simulink model "benchmark_model_2"  (R2021a)
settings: Solver=ode1  StartTime=0.0  StopTime=Tend  FixedStep=0.0001  MaxStep=0.1  MinStep=0.0001  AbsTol=0.01  EnableMultiTasking=on
values from neighbouring files (symbols this model uses):
  A1 = 0.00017774967488    [engine_data.mat]
  A2 = 740220.330082    [engine_data.mat]
  AL = [6 6.5 7 7.5 8 8.5 9 9.5 10 10.5 11 11.5 ... (33 elements, 33x1)]    [engine_data.mat]
  AM0 = 0.02884    [engine_data.mat]
  AREA = 0.00580880481649    [engine_data.mat]
  BORE = 0.086    [engine_data.mat]
  C_EGR = 1.5    [engine_data.mat]
  c_f = 800000    [engine_data.mat]
  c_T = 1    [engine_data.mat]
  CAIR = [0 0 0 0.21 0 0 0.79]    [engine_data.mat]
  cCO = 0    [engine_data.mat]
  cCO2 = 0    [engine_data.mat]
  cH2 = 0    [engine_data.mat]
  cH2O = 0    [engine_data.mat]
  cHC = 0    [engine_data.mat]
  cN2 = 0.79    [engine_data.mat]
  CO = [22.3416398376 20.8398063107 19.3759939408 17.9445472871 16.538827802 15.1528221174 13.7819470707 12.4234138404 11.076283262 9.74128071245 8.42044156849 7.11667724438 ... (33 elements, 33x1)]    [engine_data.mat]
  CO2 = [1.08016197936 1.63070203699 2.20578946805 2.80905596198 3.44329822989 4.11013545224 4.80975559522 5.54078746844 6.30033629562 7.08419123341 7.88717005398 8.70352822078 ... (33 elements, 33x1)]    [engine_data.mat]
  cO2 = 0.21    [engine_data.mat]
  DEN0 = 1.17881164668    [engine_data.mat]
  EGR_dia = 0.02    [engine_data.mat]
  EGR_sk = 0.125663706144    [engine_data.mat]
  EX_AREA = 0.00137444678595    [engine_data.mat]
  EX_M_AR = 0.0258532162804    [engine_data.mat]
  EXO = 40    [engine_data.mat]
  FD0 = 5    [engine_data.mat]
  FOM = [12 11.348 6.233 5 5.449 8.523 5]    [engine_data.mat]
  FR0 = 0    [engine_data.mat]
  FR_C1 = 305.731    [engine_data.mat]
  FR_C2 = 1.70183    [engine_data.mat]
  FR_C3 = 3188.7424    [engine_data.mat]
  FR_C4 = 0.000296028194151    [engine_data.mat]
  FR_C5 = 1.03    [engine_data.mat]
  H2 = [17.3855302766 15.0102176452 12.8820660449 10.9850020715 9.30240027035 7.81790027685 6.51548255669 5.37933989743 4.39378660966 3.5433012035 2.8127075229 2.1874445405 ... (33 elements, 33x1)]    [engine_data.mat]
  H2O = [3.81120036781 5.32559240945 6.64944794012 7.79700886885 8.78142378855 9.61507632366 10.310008356 10.8782622871 11.3320540899 11.6837509075 11.9456809954 12.1298414055 ... (33 elements, 33x1)]    [engine_data.mat]
  HC = [5481.3024964 4476.06435729 3754.34247414 3215.30411383 2799.83726136 2471.30975971 2205.97110777 1987.83348465 1805.78690133 1651.89669698 1520.35918152 1406.8402103 ... (33 elements, 33x1)]    [engine_data.mat]
  INC = 0    [engine_data.mat]
  INO = -40    [engine_data.mat]
  KET = 0.001    [engine_data.mat]
  Kex = 1.28224854645    [engine_data.mat]
  Kh = 0.00462    [engine_data.mat]
  MAS0 = 0.00471524658673    [engine_data.mat]
  MCh = 0.000588883862304    [engine_data.mat]
  MHC = 0.01383448    [engine_data.mat]
  MN2 = 0.028    [engine_data.mat]
  MO2 = 0.032    [engine_data.mat]
  MOLcylT = 0.00157069204711    [engine_data.mat]
  N2 = [54.5020363032 56.4529864816 58.2465252261 59.8999246568 61.4284172656 62.8453054261 64.1621746691 65.3891205654 66.5349581592 67.6074047194 68.6132342687 69.5584035698 ... (33 elements, 33x1)]    [engine_data.mat]
  O2 = [0.331300985803 0.293088680307 0.264743132617 0.242930742419 0.225648917415 0.211629427842 0.200034641439 0.190292592782 0.182002893523 0.174881554044 0.168729672297 0.163420998081 ... (33 elements, 33x1)]    [engine_data.mat]
  PR0 = 101324.72    [engine_data.mat]
  R150 = 157.079632679    [engine_data.mat]
  Rabs = 8.31441    [engine_data.mat]
  SPEC = [4 0.086 0.086 0.043 0.14665 14 1 0.1 0 0.5 0.005 0 ... (19 elements, 19x1)]    [engine_data.mat]
  TBORE = 0.055    [engine_data.mat]
  Tend = 120    [engine_data.mat]
  Th_HC = 0.1    [engine_data.mat]
  Th_knock = 0.401961937891    [engine_data.mat]
  THEX = [0 1 2 3 4 5 6 7 8 9 10 11 ... (721 elements, 1x721)]    [engine_data.mat]
  THIN = [0 1 2 3 4 5 6 7 8 9 10 11 ... (721 elements, 1x721)]    [engine_data.mat]
  TM0 = 298.15    [engine_data.mat]
  Tstart = 5    [engine_data.mat]
  TW0 = 353.15    [engine_data.mat]
  V_EX = 0.0001    [engine_data.mat]
  VAREX = [0 0 0 0 0 0 0 0 0 0 0 0 ... (721 elements, 1x721)]    [engine_data.mat]
  VARIN = [0 0 0 0 0 0 0 0 0 0 0 0 ... (721 elements, 1x721)]    [engine_data.mat]
  VH = 0.000499557214218    [engine_data.mat]
  VT = 3.84274780168e-05    [engine_data.mat]
  WOM = [0.01383448 0.04401 0.02801 0.032 0.002016 0.018016 0.028]    [engine_data.mat]
  y = 1.81    [engine_data.mat]
undefined symbols (not defined in the file or in its folder): DiscIntNeverNeededParam
libraries: pid_lib x3
(part 1 of 7)
settings Model: SimulationMode=accelerator  ExtModeTrigMode=oneshot  ExtModeArmWhenConnect=off  Creator=mobile  LastModifiedBy=Seb
settings SolverCC: AutoScaleAbsTol=off  ZeroCrossControl=DisableAll  AlgebraicLoopSolver=TrustRegion
settings DataIOCC: SaveFormat=Array  SignalLoggingSaveFormat=ModelDataLogs  ReturnWorkspaceOutputs=off
settings OptimizationCC: BlockReduction=off  BooleanDataType=off  ExpressionDepthLimit=2147483647  InitFltsAndDblsToZero=on  LifeSpan=inf
settings DebuggingCC: SaveWithParameterizedLinksMsg=none  UnderspecifiedInitializationDetection=Classic  MergeDetectMultiDrivingBlocksExec=none  SignalResolutionControl=TryResolveAllWithWarning  MultiTaskDSMMsg=warning  MultiTaskCondExecSysMsg=none  IntegerOverflowMsg=none  FcnCallInpInsideContextMsg=warning  StateNameClashWarn=warning  SFUnexpectedBacktrackingDiag=warning  SFNoUnconditionalDefaultTransitionDiag=warning  SFExecutionAtInitializationDiag=none  SFMachineParentedDataDiag=warning  IntegerSaturationMsg=none  ArithmeticOperatorsInVariantConditions=warning
settings HardwareCC: ProdBitPerPointer=32  ProdBitPerSizeT=32  ProdBitPerPtrDiffT=32  ProdLargestAtomicFloat=None  ProdIntDivRoundTo=Undefined  ProdEndianess=Unspecified  ProdWordSize=32  ProdHWDeviceType=32-bit Generic  TargetBitPerPointer=64  TargetBitPerSizeT=64  TargetBitPerPtrDiffT=64  TargetLongLongMode=on  TargetIntDivRoundTo=Zero  TargetEndianess=LittleEndian  TargetWordSize=64  TargetHWDeviceType=MATLAB Host  ProdEqTarget=off
settings ModelReferenceCC: PropagateSignalLabelsOutOfModel=off
settings SFSimCC: SimUseLocalCustomCode=off  CustomCodeUndefinedFunction=UseInterfaceOnly
settings RTWCC: RTWUseLocalCustomCode=off
settings CodeAppCC: StateflowObjectComments=on
settings GRTTargetCC: TargetFcnLib=ansi_tfl_tmw.mat  TargetLangStandard=C89/C90 (ANSI)  CombineOutputUpdateFcns=off  GRTInterface=on
settings ConfigComp: CovMetricSettings=dw  CovSaveCumulativeToWorkspaceVar=on  CovSaveSingleToWorkspaceVar=on  CovExternalEMLEnable=off

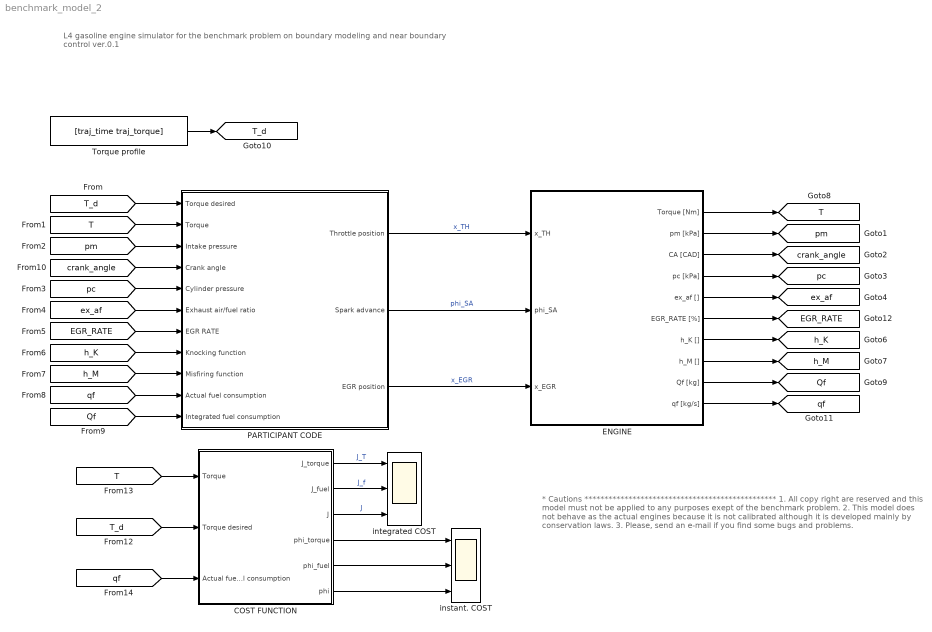
== system benchmark_model_2 ==
  note: * Cautions ************************************************
      | 1. All copy right are reserved and this model must not be applied to
      |     any purposes exept of the benchmark problem.
      | 2. This model does not behave as the actual engines because it is not
      |     calibrated although it is developed mainly by conservation laws.
      | 3. Please, send an e-mail if you find some bugs and problems.
  note: L4 gasoline engine simulator for the benchmark problem
      | on boundary modeling and near boundary control ver.0.1
  COST FUNCTION : Subsystem
  ENGINE : Subsystem
  PARTICIPANT CODE : Subsystem
  Torque profile : FromWorkspace  VariableName=[traj_time traj_torque]  SampleTime=-1  OutputAfterFinalValue=Holding final value
  instant. COST : Scope  NumInputPorts=3
  integrated COST : Scope  NumInputPorts=3
  tag scope: EGR_RATE=global, Qf=global, T=global, T_d=global, crank_angle=global, ex_af=global, h_K=global, h_M=global, pc=global, pm=global, qf=global
  wires:
  [EGR_RATE] -> PARTICIPANT CODE/7(EGR RATE)
  [h_M] -> PARTICIPANT CODE/9(Misfiring function)
  [pc] -> PARTICIPANT CODE/5(Cylinder pressure)
  [h_K] -> PARTICIPANT CODE/8(Knocking function)
  [T] -> PARTICIPANT CODE/2(Torque)
  [pm] -> PARTICIPANT CODE/3(Intake pressure)
  [qf] -> PARTICIPANT CODE/10(Actual fuel consumption)
  [ex_af] -> PARTICIPANT CODE/6(Exhaust air/fuel ratio)
  [Qf] -> PARTICIPANT CODE/11(Integrated fuel consumption)
  [T_d] -> PARTICIPANT CODE/1(Torque desired)
  Torque profile/1 -> [T_d]
  COST FUNCTION/1(J_torque) -> integrated COST/1  "J_T"
  COST FUNCTION/2(J_fuel) -> integrated COST/2  "J_f"
  COST FUNCTION/3(J) -> integrated COST/3  "J"
  [T] -> COST FUNCTION/1(Torque)
  [T_d] -> COST FUNCTION/2(Torque desired)
  [qf] -> COST FUNCTION/3(Actual fuel consumption)
  [crank_angle] -> PARTICIPANT CODE/4(Crank angle)
  PARTICIPANT CODE/1(Throttle position) -> ENGINE/1(x_TH)  "x_TH"
  PARTICIPANT CODE/2(Spark advance) -> ENGINE/2(phi_SA)  "phi_SA"
  PARTICIPANT CODE/3(EGR position) -> ENGINE/3(x_EGR)  "x_EGR"
  ENGINE/2(pm [kPa]) -> [pm]
  ENGINE/3(CA [CAD]) -> [crank_angle]
  ENGINE/4(pc [kPa]) -> [pc]
  ENGINE/5(ex_af []) -> [ex_af]
  ENGINE/7(h_K []) -> [h_K]
  ENGINE/8(h_M []) -> [h_M]
  ENGINE/1(Torque [Nm]) -> [T]
  ENGINE/9(Qf [kg]) -> [Qf]
  ENGINE/10(qf [kg/s]) -> [qf]
  ENGINE/6(EGR_RATE [%]) -> [EGR_RATE]
  COST FUNCTION/4(phi_torque) -> instant. COST/1
  COST FUNCTION/5(phi_fuel) -> instant. COST/2
  COST FUNCTION/6(phi) -> instant. COST/3

== system benchmark_model_2/COST FUNCTION ==
  Torque : Inport
  Torque desired : Inport  Port=2
  Actual fuel consumption : Inport  Port=3
  Add : Sum  Inputs=+-
  Add1 : Sum
  Add2 : Sum
  Gain : Gain  Gain=c_f
  Gain1 : Gain  Gain=c_T
  Gain2 : Gain  Gain=c_f
  Gain3 : Gain  Gain=c_T
  Integrator : Integrator
  Integrator1 : Integrator
  Math Function : Math  Operator=square  SignedPower=on  SaturateOnIntegerOverflow=on
  Product : Product
  Product1 : Product
  Step : Step  Time=Tstart  SampleTime=0
  J_torque : Outport
  J_fuel : Outport  Port=2
  J : Outport  Port=3
  phi_torque : Outport  Port=4
  phi_fuel : Outport  Port=5
  phi : Outport  Port=6
  wires:
  Torque/1 -> Add/1
  Torque desired/1 -> Add/2
  Gain/1 -> Add1/2, J_fuel/1
  Gain1/1 -> Add1/1, J_torque/1
  Math Function/1 -> Gain3/1, Integrator/1
  Integrator/1 -> Gain1/1
  Actual fuel consumption/1 -> Product/1
  Product/1 -> Gain2/1, Integrator1/1
  Step/1 -> Product1/2, Product/2
  Add/1 -> Product1/1
  Product1/1 -> Math Function/1
  Add1/1 -> J/1
  Integrator1/1 -> Gain/1
  Gain3/1 -> phi_torque/1, Add2/1
  Add2/1 -> phi/1
  Gain2/1 -> Add2/2, phi_fuel/1

== system benchmark_model_2/ENGINE ==
  x_TH : Inport
  phi_SA : Inport  Port=2
  x_EGR : Inport  Port=3
  Changing units : Subsystem
  EGR%2Lift : Fcn  Expr=u(1)/100*0.125*EGR_dia
  Ground1 : Ground
  Product : Product  RndMeth=Zero
  Terminator{,1..3} (4 alike) : Terminator
  Torq2VVT : Lookup_n-D  NumberOfTableDimensions=1  BreakpointsForDimension1=[0,6,10,20,180]  Table=[10,5,0,0,0]  RndMeth=Simplest  InputSameDT=on
  V2Vec : Constant  Value=[1 1 1 1]
  engine_s : Subsystem
  rpm : Constant  Value=1500
  Torque [Nm] : Outport
  pm [kPa] : Outport  Port=2
  CA [CAD] : Outport  Port=3
  pc [kPa] : Outport  Port=4
  ex_af [] : Outport  Port=5
  EGR_RATE [%] : Outport  Port=6
  h_K [] : Outport  Port=7
  h_M [] : Outport  Port=8
  Qf [kg] : Outport  Port=9
  qf [kg/s] : Outport  Port=10
  wires:
  engine_s/7(EGR) -> Changing units/5(C_rate)
  engine_s/6(pm) -> Changing units/4(pm)
  engine_s/10(M_HC) -> Changing units/8(RH)
  engine_s/8(R_KC) -> Changing units/6(R_KC)
  engine_s/9(B_KC) -> Changing units/7(B_KC)
  engine_s/11(TR) -> Changing units/9(torque)
  engine_s/12(Qf) -> Changing units/10(Qf)
  Ground1/1 -> engine_s/4(ECU_fi)
  engine_s/1(rps) -> Terminator/1
  engine_s/2(mt) -> Terminator1/1
  Torq2VVT/1 -> engine_s/1(ECU_VVT)
  EGR%2Lift/1 -> engine_s/5(ECU_EGR)
  Product/1 -> engine_s/3(ECU_sa)
  V2Vec/1 -> Product/2
  phi_SA/1 -> Product/1
  x_EGR/1 -> EGR%2Lift/1
  x_TH/1 -> engine_s/2(ECU_dth)
  engine_s/13(qf) -> Changing units/11(qf)
  Changing units/2(pm [kPa]) -> pm [kPa]/1
  Changing units/3(crank_angle [deg]) -> CA [CAD]/1
  Changing units/4(pc [kpa]) -> pc [kPa]/1
  Changing units/5(ex_af) -> ex_af []/1
  Changing units/12(qf [kg/s]) -> qf [kg/s]/1
  Changing units/11(Qf [kg]) -> Qf [kg]/1
  Changing units/10(T [Nm]) -> Torque [Nm]/1
  Changing units/9(h_M) -> h_M []/1
  Changing units/8(h_K) -> h_K []/1
  Changing units/6(EGR [%]) -> EGR_RATE [%]/1
  [T_d] -> Torq2VVT/1
  rpm/1 -> Changing units/12(rpm), engine_s/6(rpm)
  engine_s/4(afm) -> Changing units/2(af)
  engine_s/5(pc) -> Changing units/3(pc)
  engine_s/3(st) -> Changing units/1(st)
  Changing units/1(RPM) -> Terminator3/1
  Changing units/7(I_K) -> Terminator2/1

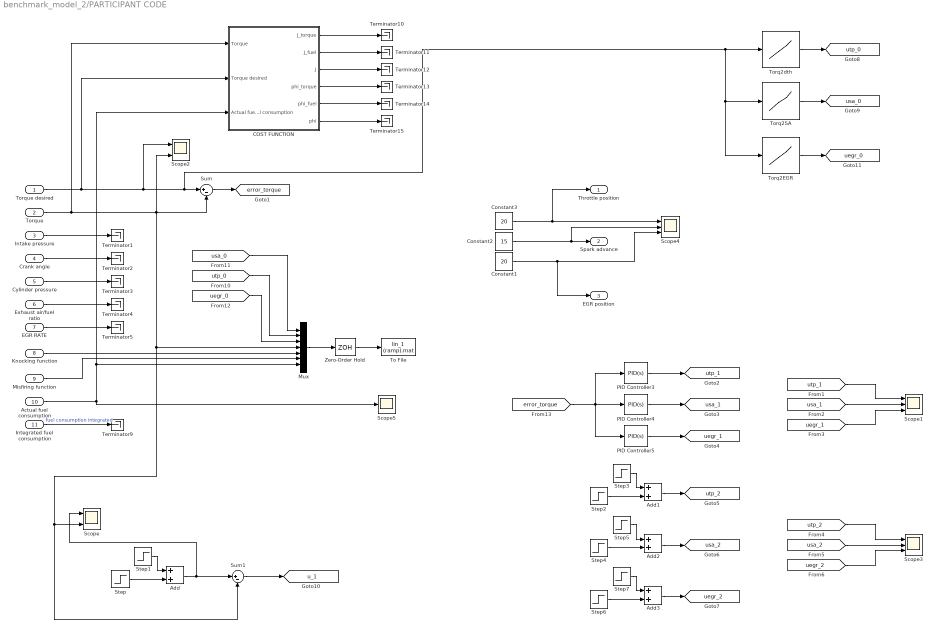
== system benchmark_model_2/PARTICIPANT CODE ==
  Torque desired : Inport
  Torque : Inport  Port=2
  Intake pressure : Inport  Port=3
  Crank angle : Inport  Port=4
  Cylinder pressure : Inport  Port=5
  Exhaust air/fuel ratio : Inport  Port=6
  EGR RATE : Inport  Port=7
  Knocking function : Inport  Port=8
  Misfiring function : Inport  Port=9
  Actual fuel consumption : Inport  Port=10
  Integrated fuel consumption : Inport  Port=11
  Add{,1..3} (4 alike) : Sum
  COST FUNCTION : Subsystem
  Constant1 : Constant  Value=20
  Constant2 : Constant  Value=15
  Constant3 : Constant  Value=20
  Mux : Mux  Inputs=7
  PID Controller3 : pid_lib/PID Controller  Controller=PID  Form=Parallel  TimeDomain=Continuous-time  UseExternalTs=off  SampleTime=-1  IntegratorMethod=Forward Euler  FilterMethod=Forward Euler  ControllerParametersSource=internal  P=0.15  I=0.75  D=0  UseFilter=on  N=100  TunerSelectOption=Transfer Function Based (PID Tuner App)  InitialConditionSource=internal  InitialConditionForIntegrator=0  InitialConditionForFilter=0  DifferentiatorICPrevScaledInput=0  ExternalReset=none  TrackingMode=off  Kt=1  LimitOutput=off  SatLimitsSource=internal  UpperSaturationLimit=inf  LowerSaturationLimit=-inf  LinearizeAsGain=on  AntiWindupMode=none  Kb=1  POutMin=[]  POutMax=[]  IOutMin=[]  IOutMax=[]  DOutMin=[]  DOutMax=[]  NOutMin=[]  NOutMax=[]  SumOutMin=[]  SumOutMax=[]  SaturationOutMin=[]  SaturationOutMax=[]  PParamMin=[]  PParamMax=[]  IParamMin=[]  IParamMax=[]  DParamMin=[]  DParamMax=[]  NParamMin=[]  NParamMax=[]  KbParamMin=[]  KbParamMax=[]  KtParamMin=[]  KtParamMax=[]  KbOutMin=[]  KbOutMax=[]  KtOutMin=[]  KtOutMax=[]  IntegratorOutMin=[]  IntegratorOutMax=[]  FilterOutMin=[]  FilterOutMax=[]  SumI1OutMin=[]  SumI1OutMax=[]  SumI2OutMin=[]  SumI2OutMax=[]  SumI3OutMin=[]  SumI3OutMax=[]  SumI4OutMin=[]  SumI4OutMax=[]  SumDOutMin=[]  SumDOutMax=[]  DifferentiatorOutMin=[]  DifferentiatorOutMax=[]  FilterDiffOutCoefMin=[]  FilterDiffOutCoefMax=[]  ReciprocalOutMin=[]  ReciprocalOutMax=[]  SumDenOutMin=[]  SumDenOutMax=[]  SumNumOutMin=[]  SumNumOutMax=[]  DivideOutMin=[]  DivideOutMax=[]  UdiffTsProdOutMin=[]  UdiffTsProdOutMax=[]  NTsProdOutMin=[]  NTsProdOutMax=[]  UintegralTsProdOutMin=[]  UintegralTsProdOutMax=[]  UngainTsProdOutMin=[]  UngainTsProdOutMax=[]  IntegratorContinuousStateAttributes=''  IntegratorStateMustResolveToSignalObject=off  IntegratorRTWStateStorageClass=Auto  FilterContinuousStateAttributes=''  FilterStateMustResolveToSignalObject=off  FilterRTWStateStorageClass=Auto  ParallelPVariant=InternalParameters  IdealPVariant=Disabled  IVariant=InternalParameters  DVariant=InternalParameters  IntegratorVariant=Continuous  SatVariant=Disabled  AWVariant=Passthrough  PCopyVariant=Disabled  TRVariant=Disabled  FdbkBlocksVariant=Forward  IdealPFdbkVariant=Disabled  SatFdbkVariant=Disabled  DerivativeFilterVariant=ContFilter  NVariant=InternalParameters  NCopyVariant=Disabled  FilterICVariant=InternalICsFilter  IntegratorICVariant=InternalICs  ExternalResetVariant=Disabled  TRSumVariant=Passthrough  SumFdbkVariant=Disabled  SumVariant=Sum_PID  TsampFilterVariant=InternalTs  TsampNgainVariant=Passthrough  TsampIntegralVariant=Passthrough  ExternalSaturationOutDataTypeStr=Inherit: Same as second input
  PID Controller4 : pid_lib/PID Controller  Controller=PID  Form=Parallel  TimeDomain=Continuous-time  UseExternalTs=off  SampleTime=-1  IntegratorMethod=Forward Euler  FilterMethod=Forward Euler  ControllerParametersSource=internal  P=0.3  I=0.1  D=0  UseFilter=on  N=100  TunerSelectOption=Transfer Function Based (PID Tuner App)  InitialConditionSource=internal  InitialConditionForIntegrator=0  InitialConditionForFilter=0  DifferentiatorICPrevScaledInput=0  ExternalReset=none  TrackingMode=off  Kt=1  LimitOutput=off  SatLimitsSource=internal  UpperSaturationLimit=inf  LowerSaturationLimit=-inf  LinearizeAsGain=on  AntiWindupMode=none  Kb=1  POutMin=[]  POutMax=[]  IOutMin=[]  IOutMax=[]  DOutMin=[]  DOutMax=[]  NOutMin=[]  NOutMax=[]  SumOutMin=[]  SumOutMax=[]  SaturationOutMin=[]  SaturationOutMax=[]  PParamMin=[]  PParamMax=[]  IParamMin=[]  IParamMax=[]  DParamMin=[]  DParamMax=[]  NParamMin=[]  NParamMax=[]  KbParamMin=[]  KbParamMax=[]  KtParamMin=[]  KtParamMax=[]  KbOutMin=[]  KbOutMax=[]  KtOutMin=[]  KtOutMax=[]  IntegratorOutMin=[]  IntegratorOutMax=[]  FilterOutMin=[]  FilterOutMax=[]  SumI1OutMin=[]  SumI1OutMax=[]  SumI2OutMin=[]  SumI2OutMax=[]  SumI3OutMin=[]  SumI3OutMax=[]  SumI4OutMin=[]  SumI4OutMax=[]  SumDOutMin=[]  SumDOutMax=[]  DifferentiatorOutMin=[]  DifferentiatorOutMax=[]  FilterDiffOutCoefMin=[]  FilterDiffOutCoefMax=[]  ReciprocalOutMin=[]  ReciprocalOutMax=[]  SumDenOutMin=[]  SumDenOutMax=[]  SumNumOutMin=[]  SumNumOutMax=[]  DivideOutMin=[]  DivideOutMax=[]  UdiffTsProdOutMin=[]  UdiffTsProdOutMax=[]  NTsProdOutMin=[]  NTsProdOutMax=[]  UintegralTsProdOutMin=[]  UintegralTsProdOutMax=[]  UngainTsProdOutMin=[]  UngainTsProdOutMax=[]  IntegratorContinuousStateAttributes=''  IntegratorStateMustResolveToSignalObject=off  IntegratorRTWStateStorageClass=Auto  FilterContinuousStateAttributes=''  FilterStateMustResolveToSignalObject=off  FilterRTWStateStorageClass=Auto  ParallelPVariant=InternalParameters  IdealPVariant=Disabled  IVariant=InternalParameters  DVariant=InternalParameters  IntegratorVariant=Continuous  SatVariant=Disabled  AWVariant=Passthrough  PCopyVariant=Disabled  TRVariant=Disabled  FdbkBlocksVariant=Forward  IdealPFdbkVariant=Disabled  SatFdbkVariant=Disabled  DerivativeFilterVariant=ContFilter  NVariant=InternalParameters  NCopyVariant=Disabled  FilterICVariant=InternalICsFilter  IntegratorICVariant=InternalICs  ExternalResetVariant=Disabled  TRSumVariant=Passthrough  SumFdbkVariant=Disabled  SumVariant=Sum_PID  TsampFilterVariant=InternalTs  TsampNgainVariant=Passthrough  TsampIntegralVariant=Passthrough  ExternalSaturationOutDataTypeStr=Inherit: Same as second input
  PID Controller5 : pid_lib/PID Controller  Controller=PID  Form=Parallel  TimeDomain=Continuous-time  UseExternalTs=off  SampleTime=-1  IntegratorMethod=Forward Euler  FilterMethod=Forward Euler  ControllerParametersSource=internal  P=0  I=0  D=0  UseFilter=on  N=100  TunerSelectOption=Transfer Function Based (PID Tuner App)  InitialConditionSource=internal  InitialConditionForIntegrator=0  InitialConditionForFilter=0  DifferentiatorICPrevScaledInput=0  ExternalReset=none  TrackingMode=off  Kt=1  LimitOutput=off  SatLimitsSource=internal  UpperSaturationLimit=inf  LowerSaturationLimit=-inf  LinearizeAsGain=on  AntiWindupMode=none  Kb=1  POutMin=[]  POutMax=[]  IOutMin=[]  IOutMax=[]  DOutMin=[]  DOutMax=[]  NOutMin=[]  NOutMax=[]  SumOutMin=[]  SumOutMax=[]  SaturationOutMin=[]  SaturationOutMax=[]  PParamMin=[]  PParamMax=[]  IParamMin=[]  IParamMax=[]  DParamMin=[]  DParamMax=[]  NParamMin=[]  NParamMax=[]  KbParamMin=[]  KbParamMax=[]  KtParamMin=[]  KtParamMax=[]  KbOutMin=[]  KbOutMax=[]  KtOutMin=[]  KtOutMax=[]  IntegratorOutMin=[]  IntegratorOutMax=[]  FilterOutMin=[]  FilterOutMax=[]  SumI1OutMin=[]  SumI1OutMax=[]  SumI2OutMin=[]  SumI2OutMax=[]  SumI3OutMin=[]  SumI3OutMax=[]  SumI4OutMin=[]  SumI4OutMax=[]  SumDOutMin=[]  SumDOutMax=[]  DifferentiatorOutMin=[]  DifferentiatorOutMax=[]  FilterDiffOutCoefMin=[]  FilterDiffOutCoefMax=[]  ReciprocalOutMin=[]  ReciprocalOutMax=[]  SumDenOutMin=[]  SumDenOutMax=[]  SumNumOutMin=[]  SumNumOutMax=[]  DivideOutMin=[]  DivideOutMax=[]  UdiffTsProdOutMin=[]  UdiffTsProdOutMax=[]  NTsProdOutMin=[]  NTsProdOutMax=[]  UintegralTsProdOutMin=[]  UintegralTsProdOutMax=[]  UngainTsProdOutMin=[]  UngainTsProdOutMax=[]  IntegratorContinuousStateAttributes=''  IntegratorStateMustResolveToSignalObject=off  IntegratorRTWStateStorageClass=Auto  FilterContinuousStateAttributes=''  FilterStateMustResolveToSignalObject=off  FilterRTWStateStorageClass=Auto  ParallelPVariant=InternalParameters  IdealPVariant=Disabled  IVariant=InternalParameters  DVariant=InternalParameters  IntegratorVariant=Continuous  SatVariant=Disabled  AWVariant=Passthrough  PCopyVariant=Disabled  TRVariant=Disabled  FdbkBlocksVariant=Forward  IdealPFdbkVariant=Disabled  SatFdbkVariant=Disabled  DerivativeFilterVariant=ContFilter  NVariant=InternalParameters  NCopyVariant=Disabled  FilterICVariant=InternalICsFilter  IntegratorICVariant=InternalICs  ExternalResetVariant=Disabled  TRSumVariant=Passthrough  SumFdbkVariant=Disabled  SumVariant=Sum_PID  TsampFilterVariant=InternalTs  TsampNgainVariant=Passthrough  TsampIntegralVariant=Passthrough  ExternalSaturationOutDataTypeStr=Inherit: Same as second input
  Scope : Scope  NumInputPorts=2
  Scope1 : Scope  NumInputPorts=3
  Scope2 : Scope  NumInputPorts=2
  Scope3 : Scope  NumInputPorts=3
  Scope4 : Scope  NumInputPorts=3
  Scope5 : Scope
  Step : Step  Time=0  After=50  SampleTime=0
  Step1 : Step  Time=15  After=30  SampleTime=0
  Step2 : Step  Time=Tend/3  Before=15  After=10  SampleTime=0
  Step3 : Step  Time=2*Tend/3  After=10  SampleTime=0
  Step4 : Step  Time=0  After=6  SampleTime=0
  Step5 : Step  Time=Tend/4  After=-4  SampleTime=0
  Step6 : Step  Time=0  After=0  SampleTime=0
  Step7 : Step  Time=3*Tend/4  After=5  SampleTime=0
  Sum : Sum  Inputs=|+-
  Sum1 : Sum  Inputs=|+-
  Terminator{1..5,9..15} (12 alike) : Terminator
  To File : ToFile  Filename=lin_1 (ramp).mat  MatrixName=u_y  SampleTime=0.1
  Torq2EGR : Lookup_n-D  NumberOfTableDimensions=1  BreakpointsForDimension1=[0,20,40,60,80,90,100,120,140,160,180,190]  Table=[0,0,2,5,10,18,25,20,14,9,5,2]  RndMeth=Simplest  InputSameDT=on
  Torq2SA : Lookup_n-D  NumberOfTableDimensions=1  BreakpointsForDimension1=[0,20,40,60,80,100,120,140,160,180]  Table=[20,25,25,25,18,14,14,14,14,14]  RndMeth=Simplest  InputSameDT=on
  Torq2dth : Lookup_n-D  NumberOfTableDimensions=1  BreakpointsForDimension1=[0,20,40,60,80,90,100,120,140,160,180,190]  Table=[7,9.2,10.8,12.6,15.4,18.2,23,25,27,29.5,35,36]  RndMeth=Simplest  InputSameDT=on
  Zero-Order Hold : ZeroOrderHold  SampleTime=0.1
  Throttle position : Outport
  Spark advance : Outport  Port=2
  EGR position : Outport  Port=3
  tag scope: error_torque=global, u_1=global, uegr_0=global, uegr_1=global, uegr_2=global, usa_0=global, usa_1=global, usa_2=global, utp_0=global, utp_1=global, utp_2=global
  wires:
  Torque desired/1 -> Scope2/1, Torq2EGR/1, Torq2SA/1, Torq2dth/1, Sum/1, COST FUNCTION/2(Torque desired)
  Integrated fuel consumption/1 -> Terminator9/1  "fuel consumption integrated"
  Torque/1 -> Sum/2, Scope/2, Sum1/2, Mux/4, Scope2/2, COST FUNCTION/1(Torque)
  Intake pressure/1 -> Terminator1/1
  Crank angle/1 -> Terminator2/1
  Cylinder pressure/1 -> Terminator3/1
  Exhaust air/fuel ratio/1 -> Terminator4/1
  EGR RATE/1 -> Terminator5/1
  Knocking function/1 -> Mux/5
  Misfiring function/1 -> Mux/6
  Actual fuel consumption/1 -> Scope5/1, COST FUNCTION/3(Actual fuel consumption), Mux/7
  COST FUNCTION/1(J_torque) -> Terminator10/1
  COST FUNCTION/2(J_fuel) -> Terminator11/1
  COST FUNCTION/3(J) -> Terminator12/1
  COST FUNCTION/4(phi_torque) -> Terminator13/1
  COST FUNCTION/5(phi_fuel) -> Terminator14/1
  COST FUNCTION/6(phi) -> Terminator15/1
  Step1/1 -> Add/1
  Step/1 -> Add/2
  Add/1 -> Scope/1, Sum1/1
  Sum1/1 -> [u_1]
  Sum/1 -> [error_torque]
  [error_torque] -> PID Controller4/1, PID Controller5/1, PID Controller3/1
  PID Controller3/1 -> [utp_1]
  PID Controller4/1 -> [usa_1]
  PID Controller5/1 -> [uegr_1]
  [uegr_1] -> Scope1/3
  [usa_1] -> Scope1/2
  [utp_1] -> Scope1/1
  Step2/1 -> Add1/2
  Step3/1 -> Add1/1
  Step5/1 -> Add2/1
  Step4/1 -> Add2/2
  Step6/1 -> Add3/2
  Add1/1 -> [utp_2]
  Add2/1 -> [usa_2]
  Add3/1 -> [uegr_2]
  Step7/1 -> Add3/1
  [utp_2] -> Scope3/1
  [usa_2] -> Scope3/2
  [uegr_2] -> Scope3/3
  Mux/1 -> Zero-Order Hold/1
  [uegr_0] -> Mux/3
  [utp_0] -> Mux/2
  [usa_0] -> Mux/1
  Torq2dth/1 -> [utp_0]
  Torq2SA/1 -> [usa_0]
  Torq2EGR/1 -> [uegr_0]
  Zero-Order Hold/1 -> To File/1
  Constant3/1 -> Throttle position/1, Scope4/1
  Constant2/1 -> Scope4/2, Spark advance/1
  Constant1/1 -> EGR position/1, Scope4/3

== system benchmark_model_2/ENGINE/Changing units ==
  st : Inport
  af : Inport  Port=2
  pc : Inport  Port=3
  pm : Inport  Port=4
  C_rate : Inport  Port=5
  R_KC : Inport  Port=6
  B_KC : Inport  Port=7
  RH : Inport  Port=8
  torque : Inport  Port=9
  Qf : Inport  Port=10
  qf : Inport  Port=11
  rpm : Inport  Port=12
  Gain : Gain  Gain=1/1000  SaturateOnIntegerOverflow=on  OutDataTypeStr=Inherit: Same as input  ParamDataTypeStr=Inherit: Same as input
  Gain2 : Gain  Gain=1.0e-3  SaturateOnIntegerOverflow=on  OutDataTypeStr=Inherit: Same as input  ParamDataTypeStr=Inherit: Same as input
  Gain3 : Gain  Gain=100  SaturateOnIntegerOverflow=on  OutDataTypeStr=Inherit: Same as input  ParamDataTypeStr=Inherit: Same as input
  select : Subsystem
  RPM : Outport
  pm [kPa] : Outport  Port=2
  crank_angle [deg] : Outport  Port=3
  pc [kpa] : Outport  Port=4
  ex_af : Outport  Port=5
  EGR [%] : Outport  Port=6
  I_K : Outport  Port=7
  h_K : Outport  Port=8
  h_M : Outport  Port=9
  T [Nm] : Outport  Port=10
  Qf [kg] : Outport  Port=11
  qf [kg/s] : Outport  Port=12
  wires:
  pm/1 -> Gain/1
  Gain/1 -> pm [kPa]/1
  pc/1 -> Gain2/1
  Gain2/1 -> pc [kpa]/1
  st/1 -> select/1(st)
  select/1(crank) -> crank_angle [deg]/1
  af/1 -> ex_af/1
  C_rate/1 -> Gain3/1
  Gain3/1 -> EGR [%]/1
  RH/1 -> h_M/1
  B_KC/1 -> h_K/1
  R_KC/1 -> I_K/1
  rpm/1 -> RPM/1
  torque/1 -> T [Nm]/1
  Qf/1 -> Qf [kg]/1
  qf/1 -> qf [kg/s]/1

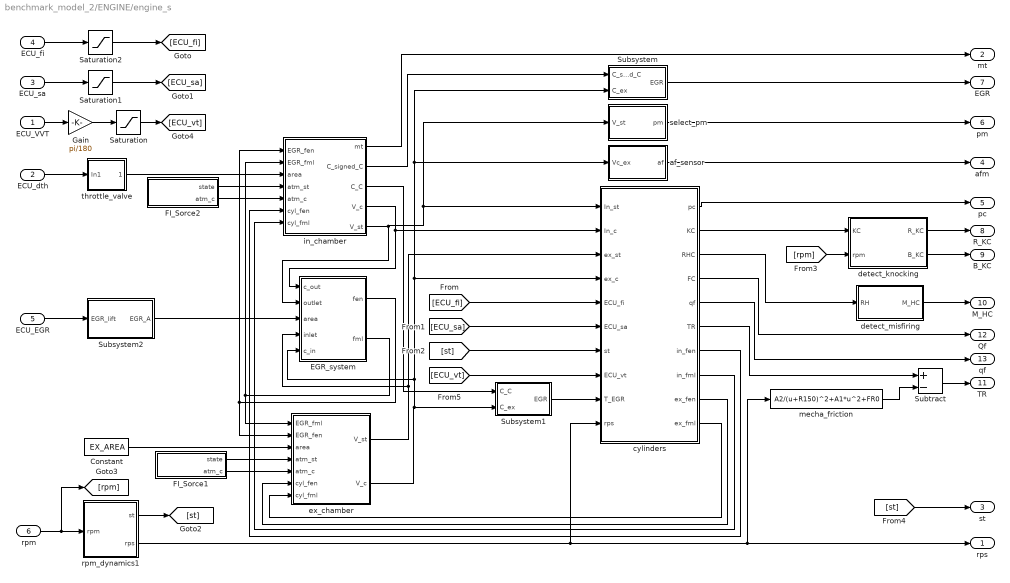
== system benchmark_model_2/ENGINE/engine_s ==
  ECU_VVT : Inport
  ECU_dth : Inport  Port=2
  ECU_sa : Inport  Port=3
  ECU_fi : Inport  Port=4
  ECU_EGR : Inport  Port=5
  rpm : Inport  Port=6
  Constant : Constant  Value=EX_AREA
  EGR_system : Subsystem
  FI_Sorce1 : Subsystem  mask(Fl_source_block){PRES=PR0, MOLC=AM0, FRDM=FD0, TEMP=TM0}
      mask prompts: PRES "Pressure"; MOLC "Mass per mol"; FRDM "Freedom"; TEMP "Temperature"
      mask init:
      | DENS=PRES/(8.31441/MOLC)/TEMP;
      | ENGY=(FRDM/2.0)*(8.31441/MOLC)*TEMP;
      mask Display: disp(' Atomspher');
  FI_Sorce2 : Subsystem  mask(Fl_source_block){PRES=PR0, MOLC=AM0, FRDM=FD0, TEMP=TM0}
      mask prompts: PRES "Pressure"; MOLC "Mass per mol"; FRDM "Freedom"; TEMP "Temperature"
      mask init:
      | DENS=PRES/(8.31441/MOLC)/TEMP;
      | ENGY=(FRDM/2.0)*(8.31441/MOLC)*TEMP;
      mask Display: disp(' Atomspher');
  Gain : Gain  Gain=pi/180
  Saturation : Saturate  UpperLimit=60*pi/180  LowerLimit=0
  Saturation1 : Saturate  UpperLimit=60  LowerLimit=-30
  Saturation2 : Saturate  UpperLimit=inf  LowerLimit=0
  Subsystem : Subsystem
  Subsystem1 : Subsystem
  Subsystem2 : Subsystem
  Subtract : Sum  Inputs=+-
  af_sensor : Subsystem
  cylinders : Subsystem
  detect_knocking : Subsystem
  detect_misfiring : Subsystem
  ex_chamber : Subsystem
  in_chamber : Subsystem
  mecha_friction : Fcn  Expr=A2/(u+R150)^2+A1*u^2+FR0
  rpm_dynamics1 : Subsystem
  select_pm : Subsystem
  throttle_valve : Subsystem
  rps : Outport
  mt : Outport  Port=2
  st : Outport  Port=3
  afm : Outport  Port=4
  pc : Outport  Port=5
  pm : Outport  Port=6
  EGR : Outport  Port=7
  R_KC : Outport  Port=8
  B_KC : Outport  Port=9
  M_HC : Outport  Port=10
  TR : Outport  Port=11
  Qf : Outport  Port=12
  qf : Outport  Port=13
  wires:
  throttle_valve/1(Out1) -> in_chamber/3(area)
  ECU_dth/1 -> throttle_valve/1(In1)
  FI_Sorce2/1(state) -> in_chamber/4(atm_st)
  in_chamber/5(V_st) -> cylinders/1(In_st), select_pm/1(V_st), EGR_system/2(outlet)
  FI_Sorce2/2(atm_c) -> in_chamber/5(atm_c)
  in_chamber/4(V_c) -> EGR_system/1(c_out), cylinders/2(In_c)
  ex_chamber/1(V_st) -> EGR_system/4(inlet), cylinders/3(ex_st)
  Constant/1 -> ex_chamber/3(area)
  cylinders/1(pc) -> pc/1
  cylinders/8(in_fml) -> in_chamber/7(cyl_fml)
  cylinders/7(in_fen) -> in_chamber/6(cyl_fen)
  cylinders/10(ex_fml) -> ex_chamber/7(cyl_fml)
  cylinders/9(ex_fen) -> ex_chamber/6(cyl_fen)
  FI_Sorce1/1(state) -> ex_chamber/4(atm_st)
  FI_Sorce1/2(atm_c) -> ex_chamber/5(atm_c)
  in_chamber/1(mt) -> mt/1
  af_sensor/1(af) -> afm/1
  ex_chamber/2(V_c) -> EGR_system/5(c_in), cylinders/4(ex_c), af_sensor/1(Vc_ex), Subsystem/2(C_ex), Subsystem1/2(C_ex)
  select_pm/1(pm) -> pm/1
  EGR_system/1(fen) -> ex_chamber/2(EGR_fen), in_chamber/1(EGR_fen)
  EGR_system/2(fml) -> ex_chamber/1(EGR_fml), in_chamber/2(EGR_fml)
  cylinders/2(KC) -> detect_knocking/1(KC)
  Subsystem/1(EGR) -> EGR/1
  in_chamber/2(C_signed_C) -> Subsystem/1(C_signed_C)
  Subsystem1/1(EGR) -> cylinders/9(T_EGR)
  in_chamber/3(C_C) -> Subsystem1/1(C_C)
  ECU_fi/1 -> Saturation2/1
  [ECU_fi] -> cylinders/5(ECU_fi)
  [ECU_sa] -> cylinders/6(ECU_sa)
  ECU_sa/1 -> Saturation1/1
  rpm/1 -> [rpm], rpm_dynamics1/1(rpm)
  [st] -> st/1
  [rpm] -> detect_knocking/2(rpm)
  detect_knocking/1(R_KC) -> R_KC/1
  detect_misfiring/1(M_HC) -> M_HC/1
  cylinders/3(RHC) -> detect_misfiring/1(RH)
  detect_knocking/2(B_KC) -> B_KC/1
  rpm_dynamics1/2(rps) -> cylinders/10(rps), mecha_friction/1, rps/1
  rpm_dynamics1/1(st) -> [st]
  [st] -> cylinders/7(st)
  ECU_VVT/1 -> Gain/1
  [ECU_vt] -> cylinders/8(ECU_vt)
  Saturation/1 -> [ECU_vt]
  Saturation1/1 -> [ECU_sa]
  Saturation2/1 -> [ECU_fi]
  ECU_EGR/1 -> Subsystem2/1(EGR_lift)
  Subsystem2/1(EGR_A) -> EGR_system/3(area)
  Gain/1 -> Saturation/1
  cylinders/6(TR) -> Subtract/1
  cylinders/4(FC) -> Qf/1
  Subtract/1 -> TR/1
  mecha_friction/1 -> Subtract/2
  cylinders/5(qf) -> qf/1

== system benchmark_model_2/PARTICIPANT CODE/COST FUNCTION ==
  Torque : Inport
  Torque desired : Inport  Port=2
  Actual fuel consumption : Inport  Port=3
  Add : Sum  Inputs=+-
  Add1 : Sum
  Add2 : Sum
  Gain : Gain  Gain=c_f
  Gain1 : Gain  Gain=c_T
  Gain2 : Gain  Gain=c_f
  Gain3 : Gain  Gain=c_T
  Integrator : Integrator
  Integrator1 : Integrator
  Math Function : Math  Operator=square  SignedPower=on  SaturateOnIntegerOverflow=on
  Product : Product
  Product1 : Product
  Step : Step  Time=Tstart  SampleTime=0
  J_torque : Outport
  J_fuel : Outport  Port=2
  J : Outport  Port=3
  phi_torque : Outport  Port=4
  phi_fuel : Outport  Port=5
  phi : Outport  Port=6
  wires:
  Torque/1 -> Add/1
  Torque desired/1 -> Add/2
  Gain/1 -> Add1/2, J_fuel/1
  Gain1/1 -> Add1/1, J_torque/1
  Math Function/1 -> Gain3/1, Integrator/1
  Integrator/1 -> Gain1/1
  Actual fuel consumption/1 -> Product/1
  Product/1 -> Gain2/1, Integrator1/1
  Step/1 -> Product1/2, Product/2
  Add/1 -> Product1/1
  Product1/1 -> Math Function/1
  Add1/1 -> J/1
  Integrator1/1 -> Gain/1
  Gain3/1 -> phi_torque/1, Add2/1
  Add2/1 -> phi/1
  Gain2/1 -> Add2/2, phi_fuel/1

== system benchmark_model_2/ENGINE/Changing units/select ==
  st : Inport
  Gain : Gain  Gain=180/pi
  Selector : Selector  InputPortWidth=4  IndexOptions=Index vector (dialog)  Indices=1  OutputSizes=[(-2)]
  crank : Outport
  wires:
  Selector/1 -> Gain/1
  Gain/1 -> crank/1
  st/1 -> Selector/1

== system benchmark_model_2/ENGINE/engine_s/EGR_system ==
  c_out : Inport
  outlet : Inport  Port=2
  area : Inport  Port=3
  inlet : Inport  Port=4
  c_in : Inport  Port=5
  Constant1 : Constant  Value=WOM
  cal_flow : MATLAB Function  TreatAsAtomicUnit=on
  fen : Outport
  fml : Outport  Port=2
  wires:
  area/1 -> cal_flow/1(area)
  cal_flow/2(fml) -> fml/1
  Constant1/1 -> cal_flow/6(WOM)
  inlet/1 -> cal_flow/2(inlet)
  c_out/1 -> cal_flow/5(c_out)
  c_in/1 -> cal_flow/3(c_in)
  outlet/1 -> cal_flow/4(outlet)
  cal_flow/1(fen) -> fen/1

== system benchmark_model_2/ENGINE/engine_s/FI_Sorce1 ==
  CO : Constant  Value=0.0
  CO2 : Constant  Value=0.0
  Dens : Constant  Value=DENS
  H2 : Constant  Value=0.0
  H2O : Constant  Value=0.0
  HC : Constant  Value=0.0
  Mux : Mux
  Mux1 : Mux  Inputs=7
  N2 : Constant  Value=0.79
  O2 : Constant  Value=0.21
  Pres : Constant  Value=PRES
  frdm : Constant  Value=FRDM
  molc : Constant  Value=MOLC
  state : Outport
  atm_c : Outport  Port=2
  wires:
  Mux1/1 -> atm_c/1
  N2/1 -> Mux1/7
  H2O/1 -> Mux1/6
  H2/1 -> Mux1/5
  O2/1 -> Mux1/4
  CO/1 -> Mux1/3
  CO2/1 -> Mux1/2
  HC/1 -> Mux1/1
  Mux/1 -> state/1
  frdm/1 -> Mux/4
  molc/1 -> Mux/3
  Pres/1 -> Mux/2
  Dens/1 -> Mux/1

== system benchmark_model_2/ENGINE/engine_s/FI_Sorce2 ==
  CO : Constant  Value=0.0
  CO2 : Constant  Value=0.0
  Dens : Constant  Value=DENS
  H2 : Constant  Value=0.0
  H2O : Constant  Value=0.0
  HC : Constant  Value=0.0
  Mux : Mux
  Mux1 : Mux  Inputs=7
  N2 : Constant  Value=0.79
  O2 : Constant  Value=0.21
  Pres : Constant  Value=PRES
  frdm : Constant  Value=FRDM
  molc : Constant  Value=MOLC
  state : Outport
  atm_c : Outport  Port=2
  wires:
  Dens/1 -> Mux/1
  Pres/1 -> Mux/2
  molc/1 -> Mux/3
  frdm/1 -> Mux/4
  Mux/1 -> state/1
  HC/1 -> Mux1/1
  CO2/1 -> Mux1/2
  CO/1 -> Mux1/3
  O2/1 -> Mux1/4
  H2/1 -> Mux1/5
  H2O/1 -> Mux1/6
  N2/1 -> Mux1/7
  Mux1/1 -> atm_c/1

== system benchmark_model_2/ENGINE/engine_s/Subsystem ==
  C_signed_C : Inport
  C_ex : Inport  Port=2
  Demux : Demux  Outputs=7
  Divide : Product  Inputs=*/
  Divide1 : Product  Inputs=/*
  Mux : Mux  Inputs=3
  Saturation : Saturate  UpperLimit=inf  LowerLimit=1.0e-16
  Saturation1 : Saturate  UpperLimit=inf  LowerLimit=0.06
  Sum of Elements : Sum  Inputs=+
  Sum of Elements1 : Sum  Inputs=+
  Terminator{,1..3} (4 alike) : Terminator
  EGR : Outport
  wires:
  C_ex/1 -> Demux/1, Sum of Elements/1
  Sum of Elements/1 -> Saturation/1
  Demux/1 -> Mux/1
  Demux/2 -> Mux/2
  Demux/3 -> Mux/3
  Mux/1 -> Sum of Elements1/1
  Sum of Elements1/1 -> Divide/1
  Demux/4 -> Terminator/1
  Demux/5 -> Terminator1/1
  Demux/6 -> Terminator2/1
  Demux/7 -> Terminator3/1
  Divide/1 -> Saturation1/1
  Saturation/1 -> Divide/2
  C_signed_C/1 -> Divide1/2
  Saturation1/1 -> Divide1/1
  Divide1/1 -> EGR/1

== system benchmark_model_2/ENGINE/engine_s/Subsystem1 ==
  C_C : Inport
  C_ex : Inport  Port=2
  Demux : Demux  Outputs=7
  Divide : Product  Inputs=*/
  Divide1 : Product  Inputs=/*
  Mux : Mux  Inputs=3
  Saturation : Saturate  UpperLimit=inf  LowerLimit=1.0e-16
  Saturation1 : Saturate  UpperLimit=inf  LowerLimit=1.0e-16
  Sum of Elements : Sum  Inputs=+
  Sum of Elements1 : Sum  Inputs=+
  Terminator{,1..3} (4 alike) : Terminator
  EGR : Outport
  wires:
  Divide1/1 -> EGR/1
  Saturation1/1 -> Divide1/1
  C_C/1 -> Divide1/2
  Saturation/1 -> Divide/2
  Divide/1 -> Saturation1/1
  Demux/7 -> Terminator3/1
  Demux/6 -> Terminator2/1
  Demux/5 -> Terminator1/1
  Demux/4 -> Terminator/1
  Sum of Elements1/1 -> Divide/1
  Mux/1 -> Sum of Elements1/1
  Demux/3 -> Mux/3
  Demux/2 -> Mux/2
  Demux/1 -> Mux/1
  Sum of Elements/1 -> Saturation/1
  C_ex/1 -> Sum of Elements/1, Demux/1

== system benchmark_model_2/ENGINE/engine_s/Subsystem2 ==
  EGR_lift : Inport
  Constant1 : Constant  Value=EGR_sk
  Product : Product
  Saturation3 : Saturate  UpperLimit=0.125*EGR_dia  LowerLimit=0
  EGR_A : Outport
  wires:
  EGR_lift/1 -> Saturation3/1
  Constant1/1 -> Product/2
  Product/1 -> EGR_A/1
  Saturation3/1 -> Product/1

== system benchmark_model_2/ENGINE/engine_s/af_sensor ==
  Vc_ex : Inport
  Constant2 : Constant  Value=[0,MO2,MO2/2,MO2,0,MO2/2,MN2]
  Constant3 : Constant  Value=[1,1,1,0,0,0,0]
  Divide : Product  Inputs=/*
  Dot Product : DotProduct  InputSameDT=on  OutDataTypeStr=Inherit: Inherit via internal rule
  Dot Product1 : DotProduct  InputSameDT=on  OutDataTypeStr=Inherit: Inherit via internal rule
  Gain : Gain  Gain=MHC
  Saturation : Saturate  UpperLimit=22  LowerLimit=6
  Saturation1 : Saturate  UpperLimit=inf  LowerLimit=1.0e-15
  af : Outport
  wires:
  Saturation/1 -> af/1
  Constant2/1 -> Dot Product1/2
  Constant3/1 -> Dot Product/2
  Gain/1 -> Saturation1/1
  Vc_ex/1 -> Dot Product/1, Dot Product1/1
  Divide/1 -> Saturation/1
  Saturation1/1 -> Divide/1
  Dot Product/1 -> Gain/1
  Dot Product1/1 -> Divide/2

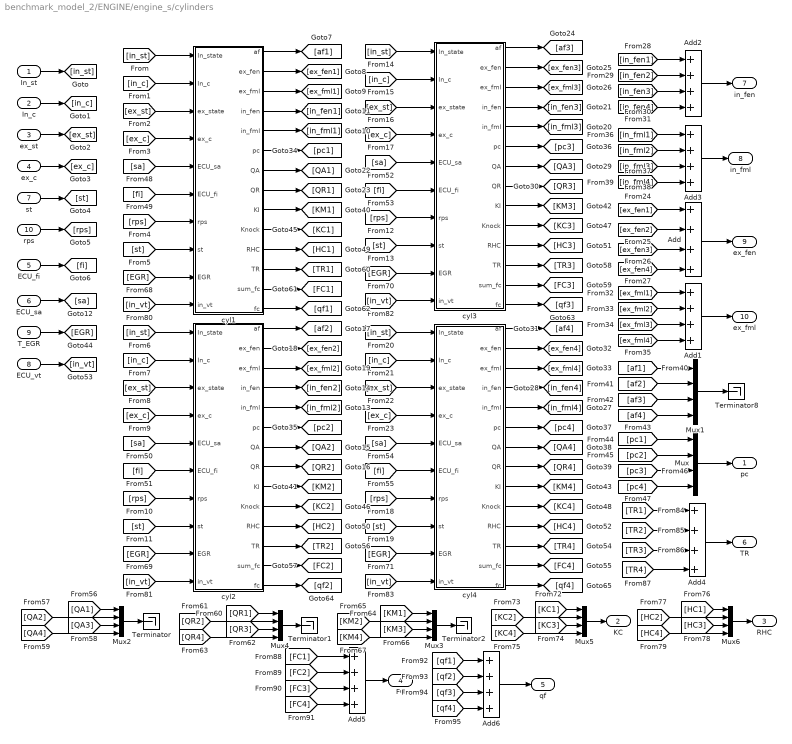
== system benchmark_model_2/ENGINE/engine_s/cylinders ==
  In_st : Inport
  In_c : Inport  Port=2
  ex_st : Inport  Port=3
  ex_c : Inport  Port=4
  ECU_fi : Inport  Port=5
  ECU_sa : Inport  Port=6
  st : Inport  Port=7
  ECU_vt : Inport  Port=8
  T_EGR : Inport  Port=9
  rps : Inport  Port=10
  Add{,1..6} (7 alike) : Sum  Inputs=++++
  Mux{,1..6} (7 alike) : Mux
  Terminator{,1..2,8} (4 alike) : Terminator
  cyl1 : Subsystem
  cyl2 : Subsystem
  cyl3 : Subsystem
  cyl4 : Subsystem
  pc : Outport
  KC : Outport  Port=2
  RHC : Outport  Port=3
  FC : Outport  Port=4
  qf : Outport  Port=5
  TR : Outport  Port=6
  in_fen : Outport  Port=7
  in_fml : Outport  Port=8
  ex_fen : Outport  Port=9
  ex_fml : Outport  Port=10
  wires:
  [pc4] -> Mux/4
  [pc3] -> Mux/3
  [pc2] -> Mux/2
  [pc1] -> Mux/1
  Mux/1 -> pc/1
  [af4] -> Mux1/4
  [af3] -> Mux1/3
  [af2] -> Mux1/2
  [af1] -> Mux1/1
  Add3/1 -> in_fml/1
  [in_fml4] -> Add3/4
  [in_fml3] -> Add3/3
  [in_fml2] -> Add3/2
  [in_fml1] -> Add3/1
  [ex_fml4] -> Add1/4
  [ex_fml3] -> Add1/3
  [ex_fml2] -> Add1/2
  [ex_fml1] -> Add1/1
  [in_fen4] -> Add2/4
  [in_fen3] -> Add2/3
  [in_fen2] -> Add2/2
  [in_fen1] -> Add2/1
  Add2/1 -> in_fen/1
  [ex_fen4] -> Add/4
  [ex_fen3] -> Add/3
  [ex_fen2] -> Add/2
  [ex_fen1] -> Add/1
  cyl1/4(in_fen) -> [in_fen1]
  cyl1/5(in_fml) -> [in_fml1]
  cyl1/3(ex_fml) -> [ex_fml1]
  cyl1/2(ex_fen) -> [ex_fen1]
  rps/1 -> [rps]
  st/1 -> [st]
  ex_c/1 -> [ex_c]
  ex_st/1 -> [ex_st]
  In_c/1 -> [in_c]
  In_st/1 -> [in_st]
  cyl1/6(pc) -> [pc1]
  Mux1/1 -> Terminator8/1
  Add1/1 -> ex_fml/1
  Add/1 -> ex_fen/1
  ECU_fi/1 -> [fi]
  ECU_sa/1 -> [sa]
  [QA1] -> Mux2/1
  [QA2] -> Mux2/2
  [QA3] -> Mux2/3
  [QA4] -> Mux2/4
  [QR1] -> Mux4/1
  [QR2] -> Mux4/2
  [QR3] -> Mux4/3
  [QR4] -> Mux4/4
  cyl1/7(QA) -> [QA1]
  cyl1/8(QR) -> [QR1]
  cyl1/9(KI) -> [KM1]
  [KM1] -> Mux3/1
  [KM2] -> Mux3/2
  [KM3] -> Mux3/3
  [KM4] -> Mux3/4
  T_EGR/1 -> [EGR]
  Mux2/1 -> Terminator/1
  Mux4/1 -> Terminator1/1
  Mux3/1 -> Terminator2/1
  cyl1/10(Knock) -> [KC1]
  [KC1] -> Mux5/1
  [KC2] -> Mux5/2
  [KC3] -> Mux5/3
  [KC4] -> Mux5/4
  Mux5/1 -> KC/1
  [HC1] -> Mux6/1
  [HC2] -> Mux6/2
  [HC3] -> Mux6/3
  [HC4] -> Mux6/4
  Mux6/1 -> RHC/1
  cyl1/11(RHC) -> [HC1]
  ECU_vt/1 -> [in_vt]
  cyl2/1(af) -> [af2]
  cyl2/2(ex_fen) -> [ex_fen2]
  cyl2/3(ex_fml) -> [ex_fml2]
  cyl2/4(in_fen) -> [in_fen2]
  cyl2/5(in_fml) -> [in_fml2]
  cyl2/6(pc) -> [pc2]
  cyl2/7(QA) -> [QA2]
  cyl2/8(QR) -> [QR2]
  cyl2/9(KI) -> [KM2]
  cyl2/10(Knock) -> [KC2]
  cyl2/11(RHC) -> [HC2]
  [in_st] -> cyl2/1(In_state)
  [in_vt] -> cyl2/10(in_vt)
  cyl3/1(af) -> [af3]
  cyl3/2(ex_fen) -> [ex_fen3]
  cyl3/3(ex_fml) -> [ex_fml3]
  cyl3/4(in_fen) -> [in_fen3]
  cyl3/5(in_fml) -> [in_fml3]
  cyl3/6(pc) -> [pc3]
  cyl3/7(QA) -> [QA3]
  cyl3/8(QR) -> [QR3]
  cyl3/9(KI) -> [KM3]
  cyl3/10(Knock) -> [KC3]
  cyl3/11(RHC) -> [HC3]
  cyl4/1(af) -> [af4]
  cyl4/2(ex_fen) -> [ex_fen4]
  cyl4/3(ex_fml) -> [ex_fml4]
  cyl4/4(in_fen) -> [in_fen4]
  cyl4/5(in_fml) -> [in_fml4]
  cyl4/6(pc) -> [pc4]
  cyl4/7(QA) -> [QA4]
  cyl4/8(QR) -> [QR4]
  cyl4/9(KI) -> [KM4]
  cyl4/10(Knock) -> [KC4]
  cyl4/11(RHC) -> [HC4]
  [in_st] -> cyl4/1(In_state)
  [in_c] -> cyl4/2(In_c)
  [ex_st] -> cyl4/3(ex_state)
  [ex_c] -> cyl4/4(ex_c)
  [sa] -> cyl4/5(ECU_sa)
  [fi] -> cyl4/6(ECU_fi)
  [rps] -> cyl4/7(rps)
  [st] -> cyl4/8(st)
  [EGR] -> cyl4/9(EGR)
  [in_vt] -> cyl4/10(in_vt)
  cyl4/12(TR) -> [TR4]
  cyl4/13(sum_fc) -> [FC4]
  [EGR] -> cyl2/9(EGR)
  [in_c] -> cyl2/2(In_c)
  [ex_st] -> cyl2/3(ex_state)
  [ex_c] -> cyl2/4(ex_c)
  [sa] -> cyl2/5(ECU_sa)
  [fi] -> cyl2/6(ECU_fi)
  [rps] -> cyl2/7(rps)
  [st] -> cyl2/8(st)
  cyl2/12(TR) -> [TR2]
  cyl2/13(sum_fc) -> [FC2]
  [in_vt] -> cyl3/10(in_vt)
  [EGR] -> cyl3/9(EGR)
  [st] -> cyl3/8(st)
  [rps] -> cyl3/7(rps)
  [fi] -> cyl3/6(ECU_fi)
  [sa] -> cyl3/5(ECU_sa)
  [ex_c] -> cyl3/4(ex_c)
  [ex_st] -> cyl3/3(ex_state)
  [in_c] -> cyl3/2(In_c)
  [in_st] -> cyl3/1(In_state)
  cyl3/12(TR) -> [TR3]
  cyl3/13(sum_fc) -> [FC3]
  [in_vt] -> cyl1/10(in_vt)
  [EGR] -> cyl1/9(EGR)
  [st] -> cyl1/8(st)
  [rps] -> cyl1/7(rps)
  [fi] -> cyl1/6(ECU_fi)
  [sa] -> cyl1/5(ECU_sa)
  [ex_c] -> cyl1/4(ex_c)
  [ex_st] -> cyl1/3(ex_state)
  [in_c] -> cyl1/2(In_c)
  [in_st] -> cyl1/1(In_state)
  cyl1/12(TR) -> [TR1]
  cyl1/13(sum_fc) -> [FC1]
  [TR1] -> Add4/1
  [TR2] -> Add4/2
  [TR3] -> Add4/3
  [TR4] -> Add4/4
  Add4/1 -> TR/1
  cyl1/1(af) -> [af1]
  cyl1/14(fc) -> [qf1]
  cyl3/14(fc) -> [qf3]
  cyl2/14(fc) -> [qf2]
  cyl4/14(fc) -> [qf4]
  [FC1] -> Add5/1
  [FC4] -> Add5/4
  [FC2] -> Add5/2
  [FC3] -> Add5/3
  Add5/1 -> FC/1
  [qf2] -> Add6/2
  [qf1] -> Add6/1
  [qf3] -> Add6/3
  [qf4] -> Add6/4
  Add6/1 -> qf/1

== system benchmark_model_2/ENGINE/engine_s/detect_knocking ==
  KC : Inport
  rpm : Inport  Port=2
  Add : Sum  Inputs=+-
  Constant : Constant  Value=Th_knock
  Divide : Product  Inputs=*/
  Relational Operator : RelationalOperator  OutDataTypeStr=boolean  RndMeth=Nearest
  Terminator : Terminator
  R_KC : Outport
  B_KC : Outport  Port=2
  wires:
  KC/1 -> Divide/1
  rpm/1 -> Divide/2
  Divide/1 -> Add/1, R_KC/1, Relational Operator/1
  Constant/1 -> Add/2, Relational Operator/2
  Add/1 -> B_KC/1
  Relational Operator/1 -> Terminator/1

== system benchmark_model_2/ENGINE/engine_s/detect_misfiring ==
  RH : Inport
  Add : Sum  Inputs=+-
  Constant1 : Constant  Value=Th_HC
  Gain4 : Gain  Gain=1e5  SaturateOnIntegerOverflow=on  OutDataTypeStr=Inherit: Same as input  ParamDataTypeStr=Inherit: Same as input
  Relational Operator1 : RelationalOperator  OutDataTypeStr=boolean  RndMeth=Nearest
  Terminator : Terminator
  M_HC : Outport
  wires:
  RH/1 -> Gain4/1
  Gain4/1 -> Relational Operator1/1, Add/1
  Constant1/1 -> Add/2, Relational Operator1/2
  Add/1 -> M_HC/1
  Relational Operator1/1 -> Terminator/1

== system benchmark_model_2/ENGINE/engine_s/ex_chamber ==
  EGR_fml : Inport
  EGR_fen : Inport  Port=2
  area : Inport  Port=3
  atm_st : Inport  Port=4
  atm_c : Inport  Port=5  PortDimensions=7
  cyl_fen : Inport  Port=6
  cyl_fml : Inport  Port=7
  Constant : Constant  Value=WOM
  In_vol : Subsystem  mask(Customized Fcn){VL=V_EX, PRE=PR0, TEMP=TM0, CAIR=CAIR, FOM=FOM, Rabs=Rabs}
      mask prompts: VL "Volume"; PRE "Pressure"; TEMP "Temperature"; CAIR "Conc. of Composition"; FOM "Degree of Freedom"
      mask help:
      | General expression block. Use "u" as the input variable name.
      | Example: sin(u[1]*exp(2.3*-u[2]))
      mask init:
      | N=PRE*VL/(Rabs*TEMP);
      | Ninit=CAIR*N;
      | Finit=sum(CAIR.*FOM);
      | Einit=Finit/2*PRE*VL;
  Terminator : Terminator
  Terminator1 : Terminator
  cal_flow : MATLAB Function  TreatAsAtomicUnit=on
  V_st : Outport
  V_c : Outport  Port=2
  wires:
  atm_c/1 -> Terminator/1
  cyl_fml/1 -> In_vol/6(in_fml)
  cyl_fen/1 -> In_vol/5(in_fen)
  cal_flow/1(fen) -> In_vol/3(out_fen)
  cal_flow/2(fml) -> In_vol/4(out_fml)
  atm_st/1 -> cal_flow/4(outlet)
  area/1 -> cal_flow/1(area)
  In_vol/2(V_state) -> cal_flow/2(inlet), V_st/1
  In_vol/3(V_c) -> V_c/1, cal_flow/5(c_out), cal_flow/3(c_in)
  EGR_fen/1 -> In_vol/1(EGR_fen)
  EGR_fml/1 -> In_vol/2(EGR_fml)
  Constant/1 -> cal_flow/6(WOM)
  In_vol/1(V_temp) -> Terminator1/1

== system benchmark_model_2/ENGINE/engine_s/in_chamber ==
  EGR_fen : Inport
  EGR_fml : Inport  Port=2
  area : Inport  Port=3
  atm_st : Inport  Port=4
  atm_c : Inport  Port=5
  cyl_fen : Inport  Port=6
  cyl_fml : Inport  Port=7
  Constant : Constant  Value=WOM
  Dot Product1 : DotProduct  InputSameDT=on  OutDataTypeStr=Inherit: Inherit via internal rule
  In_vol : Subsystem  mask(Customized Fcn){VL=0.006, PRE=PR0, TEMP=TM0, CAIR=CAIR, FOM=FOM, Rabs=Rabs}
      mask prompts: VL "Volume"; PRE "Pressure"; TEMP "Temperature"; CAIR "Conc. of Composition"; FOM "Degree of Freedom"
      mask help:
      | General expression block. Use "u" as the input variable name.
      | Example: sin(u[1]*exp(2.3*-u[2]))
      mask init:
      | N=PRE*VL/(Rabs*TEMP);
      | Ninit=[CAIR*N,0.0];
      | Finit=sum(CAIR.*FOM);
      | Einit=Finit/2*PRE*VL;
  cal_flow : MATLAB Function  TreatAsAtomicUnit=on
  mt : Outport
  C_signed_C : Outport  Port=2
  C_C : Outport  Port=3
  V_c : Outport  Port=4
  V_st : Outport  Port=5  PortDimensions=4
  wires:
  cyl_fml/1 -> In_vol/4(out_fml)
  cyl_fen/1 -> In_vol/3(out_fen)
  In_vol/3(V_c) -> cal_flow/5(c_out), V_c/1
  In_vol/2(V_state) -> cal_flow/4(outlet), V_st/1
  cal_flow/2(fml) -> In_vol/6(in_fml), Dot Product1/1
  cal_flow/1(fen) -> In_vol/5(in_fen)
  atm_c/1 -> cal_flow/3(c_in)
  atm_st/1 -> cal_flow/2(inlet)
  area/1 -> cal_flow/1(area)
  Dot Product1/1 -> mt/1
  Constant/1 -> Dot Product1/2, cal_flow/6(WOM)
  EGR_fen/1 -> In_vol/1(EGR_fen)
  EGR_fml/1 -> In_vol/2(EGR_fml)
  In_vol/1(C_signed_C) -> C_signed_C/1
  In_vol/4(C_C) -> C_C/1

== system benchmark_model_2/ENGINE/engine_s/rpm_dynamics1 ==
  rpm : Inport
  Gain : Gain  Gain=pi/30
  Int.1 with initial state : Integrator
  stroke : Subsystem
  st : Outport
  rps : Outport  Port=2
  wires:
  Int.1 with initial state/1 -> stroke/1(CA)
  Gain/1 -> rps/1, Int.1 with initial state/1
  rpm/1 -> Gain/1
  stroke/1(st(1-4)) -> st/1

== system benchmark_model_2/ENGINE/engine_s/select_pm ==
  V_st : Inport
  Selector : Selector  InputPortWidth=4  IndexOptions=Index vector (dialog)  Indices=[2]  OutputSizes=1
  pm : Outport
  wires:
  V_st/1 -> Selector/1
  Selector/1 -> pm/1

== system benchmark_model_2/ENGINE/engine_s/throttle_valve ==
  In1 : Inport
  Constant : Constant  Value=0.25*pi*TBORE^2
  Fcn : Fcn  Expr=1-cos(pi/180*u)
  Product : Product  RndMeth=Zero
  Saturation : Saturate  UpperLimit=90  LowerLimit=5.0
  Out1 : Outport
  wires:
  Saturation/1 -> Fcn/1
  In1/1 -> Saturation/1
  Fcn/1 -> Product/1
  Product/1 -> Out1/1
  Constant/1 -> Product/2

== system benchmark_model_2/ENGINE/engine_s/cylinders/cyl1 ==
  In_state : Inport
  In_c : Inport  Port=2
  ex_state : Inport  Port=3
  ex_c : Inport  Port=4
  ECU_sa : Inport  Port=5
  ECU_fi : Inport  Port=6
  rps : Inport  Port=7
  st : Inport  Port=8
  EGR : Inport  Port=9
  in_vt : Inport  Port=10
  cyl : Subsystem
  ex_valve : Subsystem
  in_valve : Subsystem
  selectors : Subsystem
  af : Outport
  ex_fen : Outport  Port=2
  ex_fml : Outport  Port=3
  in_fen : Outport  Port=4
  in_fml : Outport  Port=5
  pc : Outport  Port=6
  QA : Outport  Port=7
  QR : Outport  Port=8
  KI : Outport  Port=9
  Knock : Outport  Port=10
  RHC : Outport  Port=11
  TR : Outport  Port=12
  sum_fc : Outport  Port=13
  fc : Outport  Port=14
  wires:
  rps/1 -> cyl/7(rps), selectors/7(rps)
  ECU_fi/1 -> selectors/6(ECU_fi)
  ECU_sa/1 -> selectors/5(ECU_sa)
  st/1 -> selectors/4(st)
  In_state/1 -> in_valve/5(u_st)
  ex_state/1 -> ex_valve/1(d_st)
  cyl/1(cyl_state) -> in_valve/2(d_st), ex_valve/4(u_st)
  cyl/2(cyl_c) -> ex_valve/5(u_c), in_valve/1(d_c)
  In_c/1 -> in_valve/6(u_c)
  selectors/1(ecu) -> ex_valve/3(ecu), in_valve/3(ecu), cyl/5(ecu)
  cyl/3(pc) -> pc/1
  ex_c/1 -> ex_valve/2(d_c)
  ex_valve/1(fen) -> cyl/1(ex_fen), ex_fen/1
  ex_valve/2(fml) -> cyl/2(ex_fml), ex_fml/1
  in_valve/1(fen) -> cyl/3(in_fen), in_fen/1
  in_valve/2(fml) -> cyl/4(in_fml), selectors/1(fml), in_fml/1
  cyl/4(af) -> af/1
  selectors/2(KL) -> cyl/6(KL)
  cyl/5(QA) -> QA/1
  cyl/6(QR) -> QR/1
  cyl/7(KI) -> KI/1
  in_valve/3(fms) -> selectors/2(fms)
  EGR/1 -> cyl/8(EGR)
  cyl/8(Knock) -> Knock/1
  cyl/9(R_HC) -> RHC/1
  in_vt/1 -> selectors/3(ECU_vt), in_valve/4(in_vt)
  cyl/10(TR) -> TR/1
  selectors/3(sum_fc) -> sum_fc/1
  selectors/4(fc) -> fc/1

== system benchmark_model_2/ENGINE/engine_s/cylinders/cyl2 ==
  In_state : Inport
  In_c : Inport  Port=2
  ex_state : Inport  Port=3
  ex_c : Inport  Port=4
  ECU_sa : Inport  Port=5
  ECU_fi : Inport  Port=6
  rps : Inport  Port=7
  st : Inport  Port=8
  EGR : Inport  Port=9
  in_vt : Inport  Port=10
  cyl : Subsystem
  ex_valve : Subsystem
  in_valve : Subsystem
  selectors : Subsystem
  af : Outport
  ex_fen : Outport  Port=2
  ex_fml : Outport  Port=3
  in_fen : Outport  Port=4
  in_fml : Outport  Port=5
  pc : Outport  Port=6
  QA : Outport  Port=7
  QR : Outport  Port=8
  KI : Outport  Port=9
  Knock : Outport  Port=10
  RHC : Outport  Port=11
  TR : Outport  Port=12
  sum_fc : Outport  Port=13
  fc : Outport  Port=14
  wires:
  selectors/3(sum_fc) -> sum_fc/1
  cyl/10(TR) -> TR/1
  in_vt/1 -> in_valve/4(in_vt), selectors/3(ECU_vt)
  cyl/9(R_HC) -> RHC/1
  cyl/8(Knock) -> Knock/1
  EGR/1 -> cyl/8(EGR)
  in_valve/3(fms) -> selectors/2(fms)
  cyl/7(KI) -> KI/1
  cyl/6(QR) -> QR/1
  cyl/5(QA) -> QA/1
  selectors/2(KL) -> cyl/6(KL)
  cyl/4(af) -> af/1
  in_valve/2(fml) -> in_fml/1, selectors/1(fml), cyl/4(in_fml)
  in_valve/1(fen) -> in_fen/1, cyl/3(in_fen)
  ex_valve/2(fml) -> ex_fml/1, cyl/2(ex_fml)
  ex_valve/1(fen) -> ex_fen/1, cyl/1(ex_fen)
  ex_c/1 -> ex_valve/2(d_c)
  cyl/3(pc) -> pc/1
  selectors/1(ecu) -> cyl/5(ecu), in_valve/3(ecu), ex_valve/3(ecu)
  In_c/1 -> in_valve/6(u_c)
  cyl/2(cyl_c) -> in_valve/1(d_c), ex_valve/5(u_c)
  cyl/1(cyl_state) -> ex_valve/4(u_st), in_valve/2(d_st)
  ex_state/1 -> ex_valve/1(d_st)
  In_state/1 -> in_valve/5(u_st)
  st/1 -> selectors/4(st)
  ECU_sa/1 -> selectors/5(ECU_sa)
  ECU_fi/1 -> selectors/6(ECU_fi)
  rps/1 -> selectors/7(rps), cyl/7(rps)
  selectors/4(fc) -> fc/1
